simulink model "ControlsWithAutopilot"  (Simulink 8.5)
settings: Solver=ode45  StartTime=0.0  StopTime=10.0  RelTol=1e-3
undefined symbols (not defined in the file): ap, bias, sgn, sigbuilder_block
libraries: simulink x3
(part 1 of 2)
settings Model: Creator=mddavies  LastModifiedBy=teme
settings DataIOCC: SignalLoggingSaveFormat=Dataset
settings OptimizationCC: ExpressionDepthLimit=128
settings DebuggingCC: SolverPrmCheckMsg=warning  FcnCallInpInsideContextMsg=EnableAllAsError
settings GRTTargetCC: CombineOutputUpdateFcns=on  GRTInterface=off

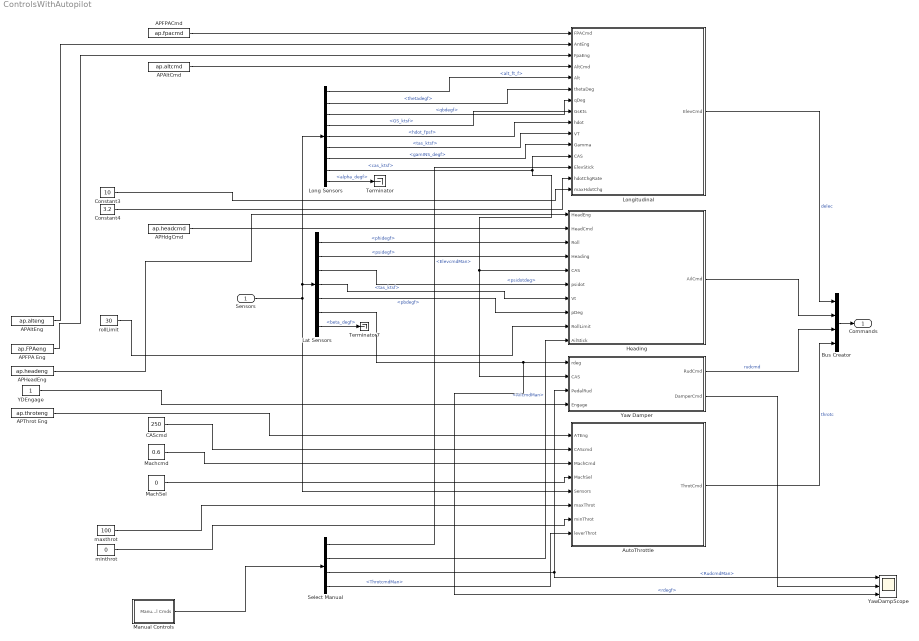
== system ControlsWithAutopilot ==
  Sensors : Inport  RequirementInfo={} %GIDa_0ce9b168_5661_42b0_b4cb_7d3faaf2df72
  APAltCmd : Constant  RequirementInfo={} %GIDa_8396ea73_c2c1_410d_8e72_0a2c2e115229  Value=ap.altcmd
  APAltEng : Constant  RequirementInfo={} %GIDa_7acdc276_5904_4f5d_a4d8_b7eafc22dcba  Value=ap.alteng  OutDataTypeStr=boolean
  APFPA Eng : Constant  RequirementInfo={} %GIDa_b6347d6f_b14e_46b8_b79f_c4482e372009  Value=ap.FPAeng  OutDataTypeStr=boolean
  "APFPACmd " : Constant  RequirementInfo={} %GIDa_f2a9802e_c9ff_44b4_9c39_101c70e3085f  Value=ap.fpacmd
  APHdgCmd : Constant  RequirementInfo={} %GIDa_ca348917_806b_4c73_b099_958ce531bbd5  Value=ap.headcmd
  APHeadEng : Constant  RequirementInfo={} %GIDa_019c8883_de5f_448b_a478_e0a40c975d97  Value=ap.headeng  OutDataTypeStr=boolean
  APThrot Eng : Constant  RequirementInfo={} %GIDa_c34ca1b2_b760_48cb_8815_eaf096d766de  Value=ap.throteng  OutDataTypeStr=boolean
  AutoThrottle : Subsystem  RequirementInfo={'other' '..\..\tcm_requirements.docx' '@Simulink_requirement_item_20' 'true' 'Auto Throttle' '' } %GIDa_9e91f8aa_3697_4e86_a547_8b20eda6b794
  Bus Creator : BusCreator  RequirementInfo={} %GIDa_5779fa34_87f2_4a60_8a6f_c75523d39478
  CAScmd : Constant  RequirementInfo={} %GIDa_47d34f1f_8d24_42cb_857b_a6284aa9b10f  Value=250
  Constant3 : Constant  RequirementInfo={} %GIDa_6046f9e1_21da_4401_862c_288f604e8689  Value=10
  Constant4 : Constant  RequirementInfo={} %GIDa_dee93be0_a932_4ef0_a207_8f7329b01ca5  Value=3.2
  Heading : Subsystem
  Lat Sensors : BusSelector  RequirementInfo={} %GIDa_c91152ab_38e9_465d_8eae_17f025af2b05  OutputSignals=phidegf,psidegf,EulerRates.psidotdeg,tas_ktsf,pbdegf,rdegf,beta_degf
  Long Sensors : BusSelector  RequirementInfo={} %GIDa_ce929a80_b046_4828_a008_4896c3439942  OutputSignals=alt_ft_f,thetadegf,qbdegf,GS_ktsf,hdot_fpsf,tas_ktsf,gamINS_degf,cas_ktsf,alpha_degf
  Longitudinal : Subsystem
  MachSel : Constant  RequirementInfo={} %GIDa_703eecf9_8ffd_4677_9df1_b11ad3ff81be  Value=0
  Machcmd : Constant  RequirementInfo={} %GIDa_a015b01e_abfd_4965_a258_bc3318cb77ef  Value=0.6
  Manual Controls : Subsystem
  Select Manual : BusSelector  RequirementInfo={} %GIDa_c52611af_90d4_4176_9d9c_eafcdc879716  OutputSignals=ElevcmdMan,AilcmdMan,RudcmdMan,ThrotcmdMan
  Terminator : Terminator
  Terminator7 : Terminator
      settings: RequirementInfo={} %GIDa_ea750fcf_3a35_4ca3_ba61_16c7ba83d83d
  YDEngage : Constant  RequirementInfo={} %GIDa_1b340559_9c71_403c_9901_bf0a93e2b9fd  SampleTime=-1
  Yaw Damper : Subsystem  RequirementInfo={'other' '..\..\tcm_requirements.docx' '@Simulink_requirement_item_19' 'true' 'Yaw Damper' '' } %GIDa_4d9fd165_a151_41ab_8542_450c342372eb
  YawDampScope : Scope  NumInputPorts=3
      settings: RequirementInfo={} %GIDa_7592f6f2_c7e8_4acc_8768_b20cb3da46c8  YMin=-5~-5~-5  YMax=5~5~5
  maxthrot : Constant  RequirementInfo={} %GIDa_230ab06c_3fb9_421e_bdda_8f032886ed67  Value=100  SampleTime=-1
  minthrot : Constant  RequirementInfo={} %GIDa_e24cf5cf_680d_403e_8bf4_a3705f2cf8ca  Value=0  SampleTime=-1
  rollLimit : Constant  RequirementInfo={} %GIDa_80188ac9_3eb7_4583_8db0_ebf7b7448de5  Value=30  SampleTime=-1
  Commands : Outport  RequirementInfo={} %GIDa_ba9bc9f0_2997_4cec_8a5a_2cb65716cddf
  wires:
  Lat Sensors/6 -> YawDampScope/3, Yaw Damper/1(rdeg)  "<rdegf>"
  AutoThrottle/1(ThrotCmd) -> Bus Creator/4  "throtc"
  Longitudinal/1(ElevCmd) -> Bus Creator/1  "delec"
  Bus Creator/1 -> Commands/1
  Heading/1(AilCmd) -> Bus Creator/2
  Sensors/1 -> Lat Sensors/1, Long Sensors/1, AutoThrottle/5(Sensors)
  Long Sensors/8 -> Yaw Damper/2(CAS), Heading/5(CAS), Longitudinal/12(CAS)  "<cas_ktsf>"
  Lat Sensors/7 -> Terminator7/1  "<beta_degf>"
  Select Manual/2 -> Heading/10(AilStick)  "<AilcmdMan>"
  Select Manual/3 -> YawDampScope/1, Yaw Damper/3(PedalRud)  "<RudcmdMan>"
  CAScmd/1 -> AutoThrottle/2(CAScmd)
  Select Manual/4 -> AutoThrottle/8(leverThrot)  "<ThrotcmdMan>"
  APAltEng/1 -> Longitudinal/2(AntEng)
  Machcmd/1 -> AutoThrottle/3(MachCmd)
  MachSel/1 -> AutoThrottle/4(MachSel)
  APHeadEng/1 -> Heading/1(HeadEng)
  APFPA Eng/1 -> Longitudinal/3(FpaEng)
  APThrot Eng/1 -> AutoThrottle/1(ATEng)
  APHdgCmd/1 -> Heading/2(HeadCmd)
  Long Sensors/9 -> Terminator/1  "<alpha_degf>"
  "APFPACmd "/1 -> Longitudinal/1(FPACmd)
  APAltCmd/1 -> Longitudinal/4(AltCmd)
  Long Sensors/1 -> Longitudinal/5(Alt)  "<alt_ft_f>"
  Long Sensors/2 -> Longitudinal/6(thetaDeg)  "<thetadegf>"
  Long Sensors/3 -> Longitudinal/7(qDeg)  "<qbdegf>"
  Long Sensors/4 -> Longitudinal/8(GsKts)  "<GS_ktsf>"
  Long Sensors/5 -> Longitudinal/9(hdot)  "<hdot_fpsf>"
  Long Sensors/6 -> Longitudinal/10(VT)  "<tas_ktsf>"
  Long Sensors/7 -> Longitudinal/11(Gamma)  "<gamINS_degf>"
  Lat Sensors/1 -> Heading/3(Roll)  "<phidegf>"
  Lat Sensors/2 -> Heading/4(Heading)  "<psidegf>"
  Lat Sensors/3 -> Heading/6(psidot)  "<psidotdeg>"
  Lat Sensors/4 -> Heading/7(Vt)  "<tas_ktsf>"
  Lat Sensors/5 -> Heading/8(pDeg)  "<pbdegf>"
  maxthrot/1 -> AutoThrottle/6(maxThrot)
  minthrot/1 -> AutoThrottle/7(minThrot)
  Select Manual/1 -> Longitudinal/13(ElevStick)  "<ElevcmdMan>"
  Yaw Damper/2(DamperCmd) -> YawDampScope/2
  Yaw Damper/1(RudCmd) -> Bus Creator/3  "rudcmd"
  Constant3/1 -> Longitudinal/15(maxHdotChg)
  Constant4/1 -> Longitudinal/14(hdotChgRate)
  YDEngage/1 -> Yaw Damper/4(Engage)
  rollLimit/1 -> Heading/9(RollLimit)
  Manual Controls/1(Manual Cmds) -> Select Manual/1

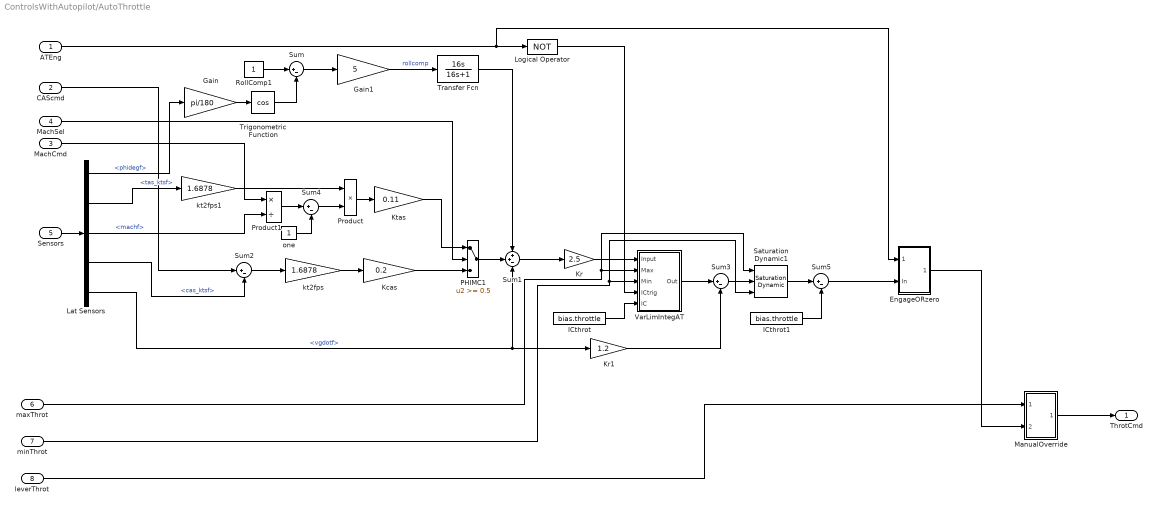
== system ControlsWithAutopilot/AutoThrottle ==
  ATEng : Inport  RequirementInfo={} %GIDa_2f45927d_6c28_4361_8173_5669474b9abd
  CAScmd : Inport  RequirementInfo={} %GIDa_92b5701d_5ed6_438c_8e94_843ad865eadf  Port=2
  MachCmd : Inport  RequirementInfo={} %GIDa_c26053c2_6b7f_4bf5_8f7d_768d0d646830  Port=3
  MachSel : Inport  RequirementInfo={} %GIDa_598b16f9_0dbe_4c96_859f_7e96536c1fb2  Port=4
  Sensors : Inport  RequirementInfo={} %GIDa_a55eff7f_fb2b_4f7a_a83b_479b402cff39  Port=5
  maxThrot : Inport  Port=6
  minThrot : Inport  Port=7
  leverThrot : Inport  Port=8
  EngageORzero : Subsystem
  Gain : Gain  RequirementInfo={} %GIDa_44ece66a_e9b1_47ae_9399_459633f82831  Gain=pi/180
  Gain1 : Gain  RequirementInfo={} %GIDa_5f70482a_3c80_415d_8392_528447a4813a  Gain=5
  ICthrot : Constant  RequirementInfo={} %GIDa_a96462ac_b28c_4fce_82e8_5e3952049bfb  Value=bias.throttle  SampleTime=-1
  ICthrot1 : Constant  RequirementInfo={} %GIDa_23dd534b_a590_436c_b15f_58e24838e8f2  Value=bias.throttle  SampleTime=-1
  Kcas : Gain  RequirementInfo={} %GIDa_1e6984b9_9479_49b0_970a_973f7c32edb7  Gain=0.2
  Kr : Gain  RequirementInfo={} %GIDa_18afb4c5_511e_47fb_85e5_bdfbcffb89de  Gain=2.5
  Kr1 : Gain  RequirementInfo={} %GIDa_9e9297b4_8c75_4533_a8dd_3891075538e5  Gain=1.2
  Ktas : Gain  RequirementInfo={} %GIDa_43c0fedf_b3e4_4e0f_a6fc_568c741b4ee2  Gain=0.11
  Lat Sensors : BusSelector  RequirementInfo={} %GIDa_4c677db3_3283_4698_82a6_69967aa56341  OutputSignals=phidegf,tas_ktsf,machf,cas_ktsf,vgdotf
  Logical Operator : Logic  RequirementInfo={} %GIDa_18e0a705_4fb5_4f14_a12b_8f6e047bc903  Operator=NOT  AllPortsSameDT=off  OutDataTypeStr=boolean
  ManualOverride : Subsystem
  PHIMC1 : Switch  RequirementInfo={} %GIDa_e2112eb0_c2db_4683_9846_bc0eb97a67f4  Threshold=0.5  SampleTime=0.02  SaturateOnIntegerOverflow=on
  Product : Product  RequirementInfo={} %GIDa_f2e51a99_89d7_4199_acd2_75b4a5a762fd  RndMeth=Zero
  Product1 : Product  RequirementInfo={} %GIDa_5c94e278_e588_4429_922d_3903b6601868  Inputs=*/  RndMeth=Zero
  RollComp1 : Constant  RequirementInfo={} %GIDa_8f810878_51f3_4d16_a407_aaec8ff4cd8a  SampleTime=-1
  Saturation Dynamic1 : simulink/Discontinuities/Saturation Dynamic  OutMin=[]  OutMax=[]  OutDataTypeStr=Inherit: Same as second input  OutDataType=sfix(16)  OutScaling=2^-10  DoSatur=off
  Sum : Sum  RequirementInfo={} %GIDa_9c88a12f_8eea_40db_a15a_aac24376aa7e  Inputs=|+-
  Sum1 : Sum  RequirementInfo={} %GIDa_fc0b036c_eb6d_4b0a_a40d_b7183183f1bc  Inputs=++-
  Sum2 : Sum  RequirementInfo={} %GIDa_95fcf8e7_99a7_46b3_9e41_77bfb2af0e6e  Inputs=|+-
  Sum3 : Sum  RequirementInfo={} %GIDa_0620e5c6_0d29_4c42_bdd5_2c680788712f  Inputs=|+-
  Sum4 : Sum  RequirementInfo={} %GIDa_a4cfd5ae_8cc7_4a4b_9229_0e28a225e0c7  Inputs=|+-
  Sum5 : Sum  RequirementInfo={} %GIDa_9cd0e9e4_7a0b_4a48_8c2a_57da4ad43678  Inputs=|+-
  Transfer Fcn : TransferFcn  RequirementInfo={} %GIDa_76b9b3a6_995f_4f78_b7a2_a7361be06aec  Numerator=[16 0]  Denominator=[16 1]
  Trigonometric Function : Trigonometry  RequirementInfo={} %GIDa_82d3b8e2_fba4_4fde_a324_6f5a5fa38b0e  Operator=cos
  VarLimIntegAT : Subsystem  RequirementInfo={} %GIDa_946bbead_442f_495f_943e_e8a8eb5a05a2
  kt2fps : Gain  RequirementInfo={} %GIDa_719dda5c_99e9_4155_8171_b1c9b5878f3a  Gain=1.6878
  kt2fps1 : Gain  RequirementInfo={} %GIDa_b06df2d8_ff63_4d20_83d9_1b3d18a391c7  Gain=1.6878
  one : Constant  RequirementInfo={} %GIDa_79530773_343c_40ed_88d6_a702a3c8b7d7  SampleTime=-1
  ThrotCmd : Outport  RequirementInfo={} %GIDa_10832092_f513_4063_bf4d_710db5c9192f
  wires:
  CAScmd/1 -> Sum2/1
  Sum2/1 -> kt2fps/1
  Sum1/1 -> Kr/1
  kt2fps/1 -> Kcas/1
  Kr/1 -> VarLimIntegAT/1(Input)
  Lat Sensors/5 -> Sum1/3, Kr1/1  "<vgdotf>"
  Kr1/1 -> Sum3/2
  Gain1/1 -> Transfer Fcn/1  "rollcomp"
  Sum/1 -> Gain1/1
  Trigonometric Function/1 -> Sum/2
  RollComp1/1 -> Sum/1
  Gain/1 -> Trigonometric Function/1
  Product1/1 -> Sum4/1
  one/1 -> Sum4/2
  Sum4/1 -> Product/2
  kt2fps1/1 -> Product/1
  Product/1 -> Ktas/1
  ICthrot/1 -> VarLimIntegAT/5(IC)
  Sum5/1 -> EngageORzero/2(In)
  ICthrot1/1 -> Sum5/2
  maxThrot/1 -> VarLimIntegAT/2(Max), Saturation Dynamic1/1
  minThrot/1 -> VarLimIntegAT/3(Min), Saturation Dynamic1/3
  VarLimIntegAT/1(Out) -> Sum3/1
  Sum3/1 -> Saturation Dynamic1/2
  Saturation Dynamic1/1 -> Sum5/1
  PHIMC1/1 -> Sum1/2
  Kcas/1 -> PHIMC1/3
  Ktas/1 -> PHIMC1/1
  Transfer Fcn/1 -> Sum1/1
  Sensors/1 -> Lat Sensors/1
  Lat Sensors/1 -> Gain/1  "<phidegf>"
  Lat Sensors/2 -> kt2fps1/1  "<tas_ktsf>"
  Lat Sensors/4 -> Sum2/2  "<cas_ktsf>"
  Logical Operator/1 -> VarLimIntegAT/4(ICtrig)
  ATEng/1 -> EngageORzero/1(Engage), Logical Operator/1
  MachSel/1 -> PHIMC1/2
  MachCmd/1 -> Product1/1
  Lat Sensors/3 -> Product1/2  "<machf>"
  leverThrot/1 -> ManualOverride/1(Man)
  ManualOverride/1(Out) -> ThrotCmd/1
  EngageORzero/1(Out) -> ManualOverride/2(Auto)

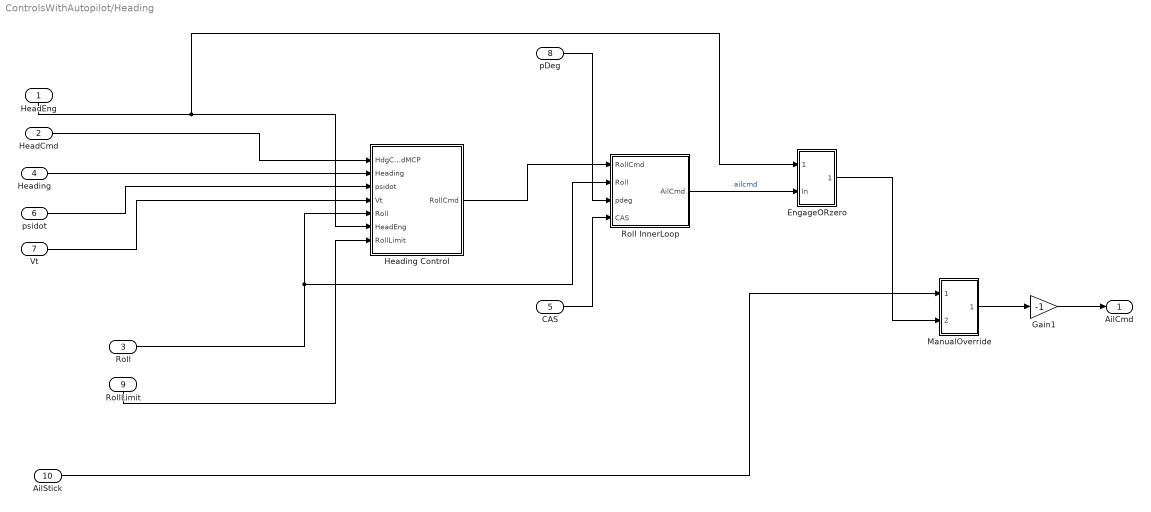
== system ControlsWithAutopilot/Heading ==
  HeadEng : Inport
  HeadCmd : Inport  Port=2
  Roll : Inport  Port=3
  Heading : Inport  Port=4
  CAS : Inport  Port=5
  psidot : Inport  Port=6
  Vt : Inport  Port=7
  pDeg : Inport  Port=8
  RollLimit : Inport  Port=9
  AilStick : Inport  Port=10
  EngageORzero : Subsystem
  Gain1 : Gain  RequirementInfo={} %GIDa_2f421c02_996e_46c9_ac2a_3c25b016b229  Gain=-1  SaturateOnIntegerOverflow=on  OutDataTypeStr=Inherit: Same as input  ParamDataTypeStr=Inherit: Same as input
  Heading Control : Subsystem  RequirementInfo={'other' '..\..\tcm_requirements.docx' '@Simulink_requirement_item_16' 'true' 'Heading Control' '' } %GIDa_911b8f78_7600_4481_9e93_a11b2a64dbe5
  ManualOverride : Subsystem
  Roll InnerLoop : Subsystem  RequirementInfo={'other' '..\..\tcm_requirements.docx' '@Simulink_requirement_item_18' 'true' 'Roll InnerLoop' '' } %GIDa_311280c1_10c2_4ab3_a776_5e785b9037f8
  AilCmd : Outport
  wires:
  pDeg/1 -> Roll InnerLoop/3(pdeg)
  Vt/1 -> Heading Control/4(Vt)
  psidot/1 -> Heading Control/3(psidot)
  Heading/1 -> Heading Control/2(Heading)
  Roll/1 -> Heading Control/5(Roll), Roll InnerLoop/2(Roll)
  Heading Control/1(RollCmd) -> Roll InnerLoop/1(RollCmd)
  Roll InnerLoop/1(AilCmd) -> EngageORzero/2(In)  "ailcmd"
  HeadCmd/1 -> Heading Control/1(HdgCmdMCP)
  HeadEng/1 -> EngageORzero/1(Engage), Heading Control/6(HeadEng)
  CAS/1 -> Roll InnerLoop/4(CAS)
  RollLimit/1 -> Heading Control/7(RollLimit)
  ManualOverride/1(Out) -> Gain1/1
  AilStick/1 -> ManualOverride/1(Man)
  Gain1/1 -> AilCmd/1
  EngageORzero/1(Out) -> ManualOverride/2(Auto)

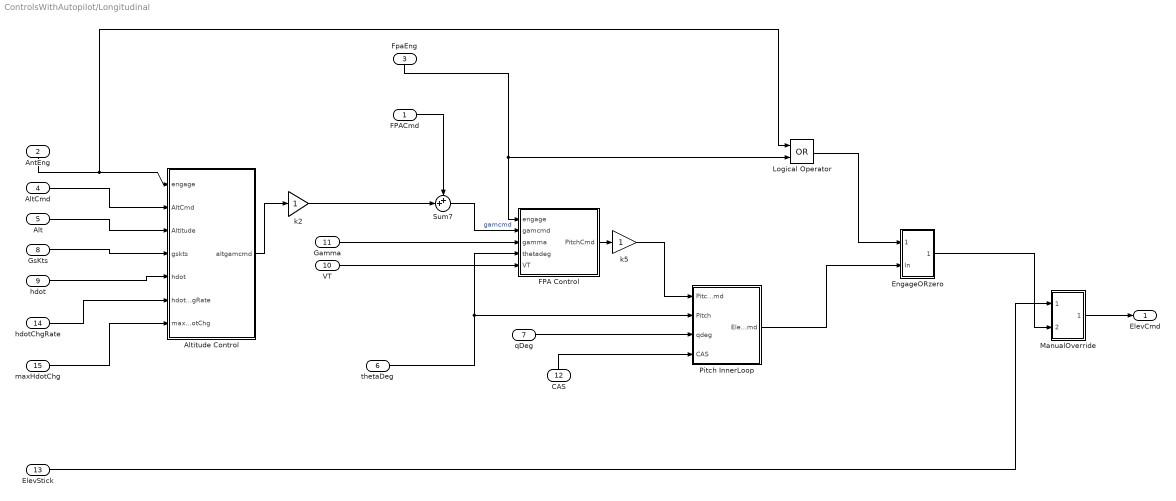
== system ControlsWithAutopilot/Longitudinal ==
  FPACmd : Inport
  AntEng : Inport  Port=2
  FpaEng : Inport  Port=3
  AltCmd : Inport  Port=4
  Alt : Inport  Port=5
  thetaDeg : Inport  Port=6
  qDeg : Inport  Port=7
  GsKts : Inport  Port=8
  hdot : Inport  Port=9
  VT : Inport  Port=10
  Gamma : Inport  Port=11
  CAS : Inport  Port=12
  ElevStick : Inport  Port=13
  hdotChgRate : Inport  Port=14
  maxHdotChg : Inport  Port=15
  Altitude Control : Subsystem  RequirementInfo={'other' '..\..\tcm_requirements.docx' '@Simulink_requirement_item_14' 'true' 'Altitude Control' '' } %GIDa_440f81f7_8b55_4c78_bea7_52c909831264
  EngageORzero : Subsystem
  FPA Control : Subsystem  RequirementInfo={'other' '..\..\tcm_requirements.docx' '@Simulink_requirement_item_15' 'true' 'FPA Control' '' } %GIDa_71e3e321_cc66_4d8a_a4f3_fd2e7f1fbaff
  Logical Operator : Logic  Operator=OR  AllPortsSameDT=off  OutDataTypeStr=boolean
  ManualOverride : Subsystem
  Pitch InnerLoop : Subsystem  RequirementInfo={'other' '..\..\tcm_requirements.docx' '@Simulink_requirement_item_17' 'true' 'Pitch InnerLoop' '' } %GIDa_fc56dd5e_d6cd_42fe_934f_e4aed2c76eb1
  Sum7 : Sum  RequirementInfo={} %GIDa_92495686_3877_4412_b19f_22e099e095ee  Inputs=++|
  k2 : Gain  RequirementInfo={} %GIDa_7e514706_5da4_4f1f_bf6c_0050dd9ce76d
  k5 : Gain  RequirementInfo={} %GIDa_b8b0ba7d_7fd3_4b03_b740_56530c3187c8
  ElevCmd : Outport
  wires:
  k2/1 -> Sum7/2
  Alt/1 -> Altitude Control/3(Altitude)
  thetaDeg/1 -> FPA Control/4(thetadeg), Pitch InnerLoop/2(Pitch)
  Gamma/1 -> FPA Control/3(gamma)
  AltCmd/1 -> Altitude Control/2(AltCmd)
  ManualOverride/1(Out) -> ElevCmd/1
  Altitude Control/1(altgamcmd) -> k2/1
  FPA Control/1(PitchCmd) -> k5/1
  hdot/1 -> Altitude Control/5(hdot)
  Sum7/1 -> FPA Control/2(gamcmd)  "gamcmd"
  qDeg/1 -> Pitch InnerLoop/3(qdeg)
  GsKts/1 -> Altitude Control/4(gskts)
  VT/1 -> FPA Control/5(VT)
  FPACmd/1 -> Sum7/1
  k5/1 -> Pitch InnerLoop/1(PitchCmd)
  FpaEng/1 -> Logical Operator/2, FPA Control/1(engage)
  CAS/1 -> Pitch InnerLoop/4(CAS)
  AntEng/1 -> Logical Operator/1, Altitude Control/1(engage)
  ElevStick/1 -> ManualOverride/1(Man)
  Pitch InnerLoop/1(ElevCmd) -> EngageORzero/2(In)
  EngageORzero/1(Out) -> ManualOverride/2(Auto)
  Logical Operator/1 -> EngageORzero/1(Engage)
  maxHdotChg/1 -> Altitude Control/7(maxHdotChg)
  hdotChgRate/1 -> Altitude Control/6(hdotChgRate)

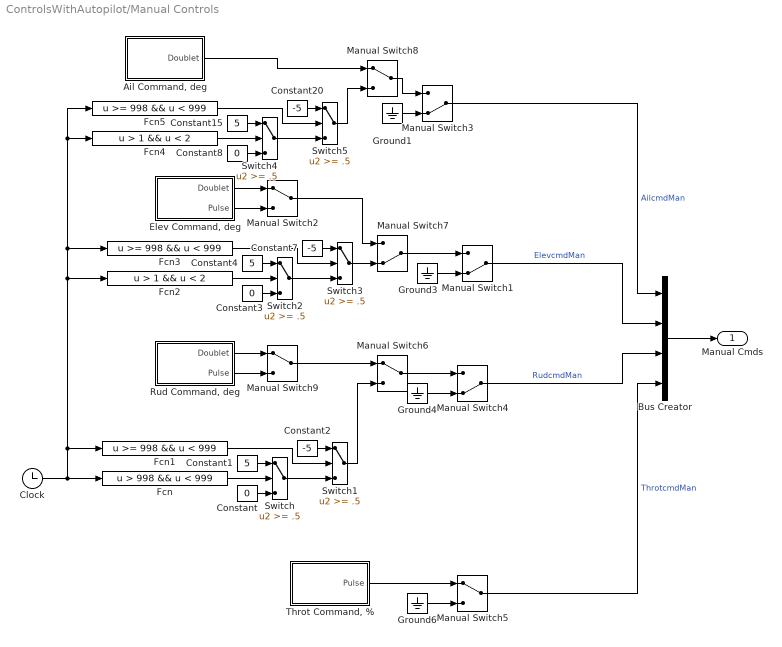
== system ControlsWithAutopilot/Manual Controls ==
  "Ail Command, deg" : Subsystem  Tag=STV Subsys  LoadFcn=sigbuilder_block('load');  StartFcn=sigbuilder_block('start');  StopFcn=sigbuilder_block('stop');  ClipboardFcn=sigbuilder_block('clipboard');  mask(Sigbuilder block){}
      mask help: Sigbuilder GUI
      mask init:
      | if ~strcmp(get_param(bdroot(gcbh),'SimulationStatus'),'stopped') tuvar = sigbuilder_block('maskInit'); end
      settings: CopyFcn=sigbuilder_block('copy');  DeleteFcn=sigbuilder_block('delete');  ModelCloseFcn=sigbuilder_block('modelClose');  PreSaveFcn=sigbuilder_block('preSave');  PauseFcn=sigbuilder_block('pause')  ContinueFcn=sigbuilder_block('continue')  NameChangeFcn=sigbuilder_block('namechange');  OpenFcn=sigbuilder_block('open',[20.16 261.12 550.08 400.32 ]);  CloseFcn=sigbuilder_block('close');
      mask Display: plot(0,0,100,100,[10,10,40,40,10],[80,20,20,80,80],[40,10],[50,50], [40,27,10],[65,72,56],[40,25,25,10],[28,28,43,43]);
  Bus Creator : BusCreator
  Clock : Clock
  Constant : Constant  Value=0
  Constant1 : Constant  Value=5
  Constant15 : Constant  Value=5
  Constant2 : Constant  Value=-5
  Constant20 : Constant  Value=-5
  Constant3 : Constant  Value=0
  Constant4 : Constant  Value=5
  Constant7 : Constant  Value=-5
  Constant8 : Constant  Value=0
  "Elev Command, deg" : Subsystem  Tag=STV Subsys  LoadFcn=sigbuilder_block('load');  StartFcn=sigbuilder_block('start');  StopFcn=sigbuilder_block('stop');  ClipboardFcn=sigbuilder_block('clipboard');  mask(Sigbuilder block){}
      mask help: Sigbuilder GUI
      mask init:
      | if ~strcmp(get_param(bdroot(gcbh),'SimulationStatus'),'stopped') tuvar = sigbuilder_block('maskInit'); end
      settings: CopyFcn=sigbuilder_block('copy');  DeleteFcn=sigbuilder_block('delete');  ModelCloseFcn=sigbuilder_block('modelClose');  PreSaveFcn=sigbuilder_block('preSave');  PauseFcn=sigbuilder_block('pause')  ContinueFcn=sigbuilder_block('continue')  NameChangeFcn=sigbuilder_block('namechange');  OpenFcn=sigbuilder_block('open',[550.08 198.72 550.08 400.32 ]);  CloseFcn=sigbuilder_block('close');
      mask Display: plot(0,0,100,100,[10,10,40,40,10],[80,20,20,80,80],[40,10],[50,50], [40,27,10],[65,72,56],[40,25,25,10],[28,28,43,43]);
  Fcn : Fcn  Expr=u > 998 && u < 999
  Fcn1 : Fcn  Expr=u >= 998 && u < 999
  Fcn2 : Fcn  Expr=u > 1 && u < 2
  Fcn3 : Fcn  Expr=u >= 998 && u < 999
  Fcn4 : Fcn  Expr=u > 1 && u < 2
  Fcn5 : Fcn  Expr=u >= 998 && u < 999
  Ground{1,3..4,6} (4 alike) : Ground
  Manual Switch{1,3..4,7} (4 alike) : ManualSwitch  CurrentSetting=0
  Manual Switch{2,5..6,8..9} (5 alike) : ManualSwitch
  "Rud Command, deg" : Subsystem  Tag=STV Subsys  LoadFcn=sigbuilder_block('load');  StartFcn=sigbuilder_block('start');  StopFcn=sigbuilder_block('stop');  ClipboardFcn=sigbuilder_block('clipboard');  mask(Sigbuilder block){}
      mask help: Sigbuilder GUI
      mask init:
      | if ~strcmp(get_param(bdroot(gcbh),'SimulationStatus'),'stopped') tuvar = sigbuilder_block('maskInit'); end
      settings: CopyFcn=sigbuilder_block('copy');  DeleteFcn=sigbuilder_block('delete');  ModelCloseFcn=sigbuilder_block('modelClose');  PreSaveFcn=sigbuilder_block('preSave');  PauseFcn=sigbuilder_block('pause')  ContinueFcn=sigbuilder_block('continue')  NameChangeFcn=sigbuilder_block('namechange');  OpenFcn=sigbuilder_block('open',[437.6 199.2 550.4 400 ]);  CloseFcn=sigbuilder_block('close');
      mask Display: plot(0,0,100,100,[10,10,40,40,10],[80,20,20,80,80],[40,10],[50,50], [40,27,10],[65,72,56],[40,25,25,10],[28,28,43,43]);
  Switch{,1..5} (6 alike) : Switch  Threshold=.5
  "Throt Command, %" : Subsystem  Tag=STV Subsys  LoadFcn=sigbuilder_block('load');  StartFcn=sigbuilder_block('start');  StopFcn=sigbuilder_block('stop');  ClipboardFcn=sigbuilder_block('clipboard');  mask(Sigbuilder block){}
      mask help: Sigbuilder GUI
      mask init:
      | if ~strcmp(get_param(bdroot(gcbh),'SimulationStatus'),'stopped') tuvar = sigbuilder_block('maskInit'); end
      settings: CopyFcn=sigbuilder_block('copy');  DeleteFcn=sigbuilder_block('delete');  ModelCloseFcn=sigbuilder_block('modelClose');  PreSaveFcn=sigbuilder_block('preSave');  PauseFcn=sigbuilder_block('pause')  ContinueFcn=sigbuilder_block('continue')  NameChangeFcn=sigbuilder_block('namechange');  OpenFcn=sigbuilder_block('open',[436.656 201.841 549.567 399.685 ]);  CloseFcn=sigbuilder_block('close');
      mask Display: plot(0,0,100,100,[10,10,40,40,10],[80,20,20,80,80],[40,10],[50,50], [40,27,10],[65,72,56],[40,25,25,10],[28,28,43,43]);
  Manual Cmds : Outport
  wires:
  Ground1/1 -> Manual Switch3/2
  Ground3/1 -> Manual Switch1/2
  "Elev Command, deg"/1(Doublet) -> Manual Switch2/1
  "Elev Command, deg"/2(Pulse) -> Manual Switch2/2
  Ground4/1 -> Manual Switch4/2
  Ground6/1 -> Manual Switch5/2
  "Throt Command, %"/1(Pulse) -> Manual Switch5/1
  Fcn/1 -> Switch/2
  Constant1/1 -> Switch/1
  Constant/1 -> Switch/3
  Switch/1 -> Switch1/3
  Constant2/1 -> Switch1/1
  Fcn1/1 -> Switch1/2
  Clock/1 -> Fcn/1, Fcn1/1, Fcn2/1, Fcn3/1, Fcn5/1, Fcn4/1
  Manual Switch6/1 -> Manual Switch4/1
  Switch1/1 -> Manual Switch6/2
  Fcn2/1 -> Switch2/2
  Constant4/1 -> Switch2/1
  Constant3/1 -> Switch2/3
  Switch2/1 -> Switch3/3
  Constant7/1 -> Switch3/1
  Fcn3/1 -> Switch3/2
  Manual Switch7/1 -> Manual Switch1/1
  Switch3/1 -> Manual Switch7/2
  Manual Switch2/1 -> Manual Switch7/1
  Fcn4/1 -> Switch4/2
  Constant15/1 -> Switch4/1
  Constant8/1 -> Switch4/3
  Switch4/1 -> Switch5/3
  Constant20/1 -> Switch5/1
  Fcn5/1 -> Switch5/2
  Manual Switch8/1 -> Manual Switch3/1
  Switch5/1 -> Manual Switch8/2
  "Ail Command, deg"/1(Doublet) -> Manual Switch8/1
  Manual Switch3/1 -> Bus Creator/1  "AilcmdMan"
  Manual Switch1/1 -> Bus Creator/2  "ElevcmdMan"
  Manual Switch4/1 -> Bus Creator/3  "RudcmdMan"
  Manual Switch5/1 -> Bus Creator/4  "ThrotcmdMan"
  Bus Creator/1 -> Manual Cmds/1
  "Rud Command, deg"/1(Doublet) -> Manual Switch9/1
  "Rud Command, deg"/2(Pulse) -> Manual Switch9/2
  Manual Switch9/1 -> Manual Switch6/1

== system ControlsWithAutopilot/Yaw Damper ==
  rdeg : Inport  RequirementInfo={} %GIDa_aab456ca_baa8_40be_af7c_3007e2406789
  CAS : Inport  RequirementInfo={} %GIDa_ffc3df4d_90ed_429c_9905_ba1d5e1c6104  Port=2
  PedalRud : Inport  Port=3
  Engage : Inport  Port=4
  EngageORzero : Subsystem
  Kcas : Lookup  RequirementInfo={} %GIDa_a54aaa82_92c8_4b54_937a_3aadc5cc777a  InputValues=[0 120 350 500]  Table=[1.0 1.0 0.3 0.3]
  Kr : Gain  RequirementInfo={} %GIDa_e1600aee_198d_416e_b040_c3f06ae50aaa  Gain=1.25
  ManualOverride : Subsystem
  Product : Product  RequirementInfo={} %GIDa_b93a6279_44c9_4030_b746_3332e584ca8b  RndMeth=Zero
  YD_wo : TransferFcn  RequirementInfo={} %GIDa_e4ecddaf_b3d8_4a89_aabe_57315209a16f  Numerator=[1 0]  Denominator=[1 10]
  RudCmd : Outport  RequirementInfo={} %GIDa_5d934514_ad75_43c8_8562_5e4d07d2a065
  DamperCmd : Outport  Port=2
  wires:
  rdeg/1 -> Kr/1
  CAS/1 -> Kcas/1
  Kcas/1 -> Product/2
  ManualOverride/1(Out) -> RudCmd/1
  Kr/1 -> YD_wo/1
  YD_wo/1 -> Product/1
  EngageORzero/1(Out) -> ManualOverride/2(Auto), DamperCmd/1
  PedalRud/1 -> ManualOverride/1(Man)
  Engage/1 -> EngageORzero/1(Engage)
  Product/1 -> EngageORzero/2(In)

== system ControlsWithAutopilot/AutoThrottle/EngageORzero ==
  Engage : Inport
  In : Inport  Port=2
  Logical Operator5 : Logic  RequirementInfo={} %GIDa_13e72d9c_1630_4494_8181_04ea596767a9  AllPortsSameDT=off  OutDataTypeStr=boolean
  Switch1 : Switch  RequirementInfo={} %GIDa_d89bdcfc_1e33_494f_b3fe_e13e317b4b5d  Threshold=0.5
  zero10 : Constant  RequirementInfo={} %GIDa_d1e784f7_2146_48f6_874a_0add9f175ac2
  zero9 : Constant  RequirementInfo={} %GIDa_df8b3a8b_00d1_4891_87af_e83379ed0682  Value=0
  Out : Outport
  wires:
  Engage/1 -> Logical Operator5/1
  zero10/1 -> Logical Operator5/2
  zero9/1 -> Switch1/3
  In/1 -> Switch1/1
  Logical Operator5/1 -> Switch1/2
  Switch1/1 -> Out/1

== system ControlsWithAutopilot/AutoThrottle/ManualOverride ==
  Man : Inport
  Auto : Inport  Port=2
  Switch1 : Switch  RequirementInfo={} %GIDa_99412258_89e8_4c84_a7a6_8adb3817b9de  Criteria=u2 ~= 0  Threshold=0.5
  Out : Outport
  wires:
  Man/1 -> Switch1/3, Switch1/2
  Auto/1 -> Switch1/1
  Switch1/1 -> Out/1

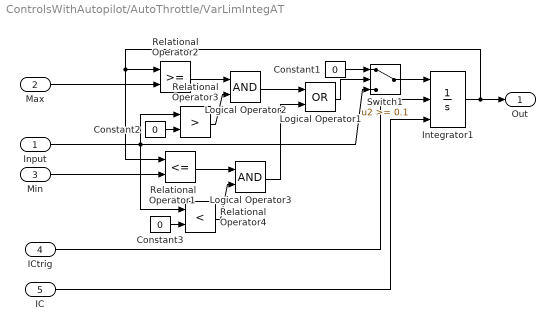
== system ControlsWithAutopilot/AutoThrottle/VarLimIntegAT ==
  Input : Inport  RequirementInfo={} %GIDa_91b38f96_ed38_45a6_8bb9_ff3fb81525df
  Max : Inport  RequirementInfo={} %GIDa_5200ce52_bb44_458c_9945_e382c2e773b4  Port=2
  Min : Inport  RequirementInfo={} %GIDa_600874e9_d5fd_4de5_b948_9284e9d56639  Port=3
  ICtrig : Inport  RequirementInfo={} %GIDa_af678c0a_424b_44b8_aa3a_3f303d846e8e  Port=4
  IC : Inport  RequirementInfo={} %GIDa_872b1a96_8436_4d34_8580_74ad3366301d  Port=5
  Constant1 : Constant  RequirementInfo={} %GIDa_bf704cc0_6bc9_4624_9fa4_e77befe43ee9  Value=0  SampleTime=-1
  Constant2 : Constant  RequirementInfo={} %GIDa_7032ed75_2ad3_41e5_9584_0891c369141c  Value=0  SampleTime=-1
  Constant3 : Constant  RequirementInfo={} %GIDa_f4367f96_4d82_41b7_8e43_0c6cec23a023  Value=0  SampleTime=-1
  Integrator1 : Integrator  RequirementInfo={} %GIDa_d4336f3d_c52f_4cf1_85ef_86b185e703b9  ExternalReset=level  InitialConditionSource=external
  Logical Operator1 : Logic  RequirementInfo={} %GIDa_53e2ecf2_1671_4b86_a4e6_7e9f03594f4a  Operator=OR
  Logical Operator2 : Logic  RequirementInfo={} %GIDa_f9639a17_73a7_4a19_b9c3_2b3e1bcf1152
  Logical Operator3 : Logic  RequirementInfo={} %GIDa_53705a9e_f0e6_4df8_b74a_51dda5b71ea0
  Relational Operator1 : RelationalOperator  RequirementInfo={} %GIDa_85cee0a0_d47b_41e2_b8dd_f48b296f5cf4  Operator=<=  InputSameDT=on
  Relational Operator2 : RelationalOperator  RequirementInfo={} %GIDa_74942223_cbc1_42b5_8e5e_e6b9112f9130  InputSameDT=on
  Relational Operator3 : RelationalOperator  RequirementInfo={} %GIDa_ea1202bb_7a42_4314_84fa_c36aa79c966a  Operator=>  InputSameDT=on
  Relational Operator4 : RelationalOperator  RequirementInfo={} %GIDa_c9e3adfb_bd3d_4cfe_9bd6_4a3fd1707fe2  Operator=<  InputSameDT=on
  Switch1 : Switch  RequirementInfo={} %GIDa_ed603307_5c4b_4569_8f05_95ce39b1df88  Threshold=0.1  SaturateOnIntegerOverflow=on  InputSameDT=on
  Out : Outport  RequirementInfo={} %GIDa_a7cb998d_eb28_45ce_8ac9_f1554f32fe4e
  wires:
  IC/1 -> Integrator1/3
  ICtrig/1 -> Integrator1/2
  Min/1 -> Relational Operator1/2
  Max/1 -> Relational Operator2/2
  Constant3/1 -> Relational Operator4/2
  Input/1 -> Switch1/3, Relational Operator3/1, Relational Operator4/1
  Logical Operator3/1 -> Logical Operator1/2
  Relational Operator4/1 -> Logical Operator3/2
  Relational Operator1/1 -> Logical Operator3/1
  Constant2/1 -> Relational Operator3/2
  Logical Operator2/1 -> Logical Operator1/1
  Relational Operator3/1 -> Logical Operator2/2
  Relational Operator2/1 -> Logical Operator2/1
  Logical Operator1/1 -> Switch1/2
  Integrator1/1 -> Relational Operator2/1, Relational Operator1/1, Out/1
  Switch1/1 -> Integrator1/1
  Constant1/1 -> Switch1/1

== system ControlsWithAutopilot/Heading/EngageORzero ==
  Engage : Inport
  In : Inport  Port=2
  Logical Operator5 : Logic  RequirementInfo={} %GIDa_7add67f6_200e_4459_8afc_a50a3802c341  AllPortsSameDT=off  OutDataTypeStr=boolean
  Switch1 : Switch  RequirementInfo={} %GIDa_a1777089_6daf_41d2_9e69_9356c4782e25  Threshold=0.5
  zero10 : Constant  RequirementInfo={} %GIDa_d889400f_b153_4cfc_a180_15b84145f1e0
  zero9 : Constant  RequirementInfo={} %GIDa_9027fd24_3b48_4acd_a774_517fb1aa3516  Value=0
  Out : Outport
  wires:
  Engage/1 -> Logical Operator5/1
  zero10/1 -> Logical Operator5/2
  zero9/1 -> Switch1/3
  In/1 -> Switch1/1
  Logical Operator5/1 -> Switch1/2
  Switch1/1 -> Out/1

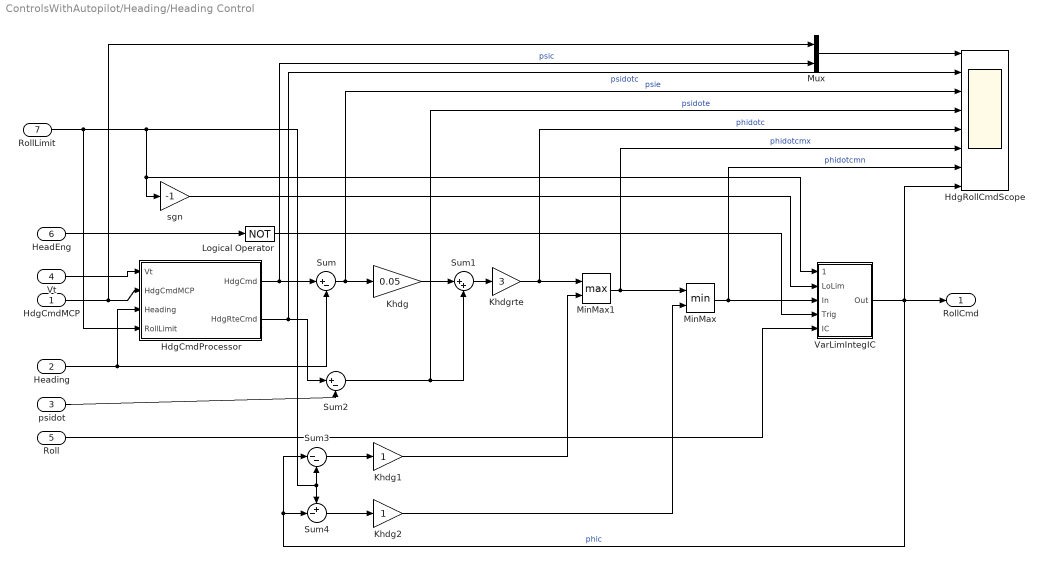
== system ControlsWithAutopilot/Heading/Heading Control ==
  HdgCmdMCP : Inport  RequirementInfo={} %GIDa_afcd05d1_a9dc_45a7_a8f8_7136ccc61726
  Heading : Inport  RequirementInfo={} %GIDa_19b80fe4_d265_482c_b709_18db80a7cdf3  Port=2
  psidot : Inport  RequirementInfo={} %GIDa_e421e82d_0cc7_4ad7_ac7a_9fb430d189d5  Port=3
  Vt : Inport  RequirementInfo={} %GIDa_9daf3e20_e00e_4f36_b534_d9747a241338  Port=4
  Roll : Inport  RequirementInfo={} %GIDa_8629ba77_a751_4097_af53_617eaa1017be  Port=5
  HeadEng : Inport  RequirementInfo={} %GIDa_dadb1310_2bf4_48cf_8970_85174d784ee3  Port=6
  RollLimit : Inport  Port=7
  HdgCmdProcessor : Subsystem  RequirementInfo={} %GIDa_3cb77e5f_f630_4f22_88a8_7528bfceb83f
  HdgRollCmdScope : Scope  NumInputPorts=8
      settings: RequirementInfo={} %GIDa_5fbe2135_fdf1_4f64_a179_faa1710ae21e  YMin=-30~-30~-10~-10~-4~-10~0~-5  YMax=30~30~10~10~4~10~1~5  SaveName=ScopeData7
  Khdg : Gain  RequirementInfo={} %GIDa_abf81b08_c210_4343_b4da_5a7e229caeb6  Gain=0.05
  Khdg1 : Gain  RequirementInfo={} %GIDa_7a7a35ca_24a5_4d20_bc30_55deea16462c
  Khdg2 : Gain  RequirementInfo={} %GIDa_57191899_7ee5_4454_897a_7009651ed5fb
  Khdgrte : Gain  RequirementInfo={} %GIDa_bcc6a420_18f3_43f0_aaa1_aaa1bbf90f64  Gain=3
  Logical Operator : Logic  RequirementInfo={} %GIDa_5ad405ac_0a88_4b96_aa0e_75483351ee25  Operator=NOT  AllPortsSameDT=off  OutDataTypeStr=boolean
  MinMax : MinMax  RequirementInfo={} %GIDa_4b9381d8_eb85_418b_a975_85846d5ca8c2  Inputs=2
  MinMax1 : MinMax  RequirementInfo={} %GIDa_b40e082d_0fb2_4088_baf4_e9a71be9bcc1  Function=max  Inputs=2
  Mux : Mux  RequirementInfo={} %GIDa_0e83f6c6_ae04_43dd_95fe_a79ec32b40e2  Inputs=2
  Sum : Sum  RequirementInfo={} %GIDa_b89885fc_f86c_4a50_8ce5_47d0488bdc1c  Inputs=|+-
  Sum1 : Sum  RequirementInfo={} %GIDa_40ec6862_b1f8_4f97_ae14_1eadabbceb30  Inputs=|++
  Sum2 : Sum  RequirementInfo={} %GIDa_307d6880_3ab8_4deb_90e0_d68f11d87c85  Inputs=|+-
  Sum3 : Sum  RequirementInfo={} %GIDa_ebb8b765_7f4a_435f_be61_680d3199141b  Inputs=|--
  Sum4 : Sum  RequirementInfo={} %GIDa_05638559_562a_476e_9e4c_91124434a43b  Inputs=+-|
  VarLimIntegIC : Subsystem  RequirementInfo={} %GIDa_7da7eaf5_9731_498e_9aad_b41279918004
  sgn : Gain  RequirementInfo={} %GIDa_84e2dc00_f2e5_41f4_89ce_c9fef234974f  Gain=-1
  RollCmd : Outport  RequirementInfo={} %GIDa_aa862f7f_5d4e_408f_b8c4_26b4ce96fbda
  wires:
  Heading/1 -> Sum/2, HdgCmdProcessor/3(Heading)
  HdgCmdProcessor/1(HdgCmd) -> Sum/1, Mux/2  "psic"
  Sum/1 -> Khdg/1, HdgRollCmdScope/3  "psie"
  Khdg/1 -> Sum1/1
  Sum2/1 -> Sum1/2, HdgRollCmdScope/4  "psidote"
  HdgCmdProcessor/2(HdgRteCmd) -> Sum2/1, HdgRollCmdScope/2  "psidotc"
  psidot/1 -> Sum2/2
  Vt/1 -> HdgCmdProcessor/1(Vt)
  HdgCmdMCP/1 -> HdgCmdProcessor/2(HdgCmdMCP), Mux/1
  VarLimIntegIC/1(Out) -> RollCmd/1, Sum3/1, Sum4/2, HdgRollCmdScope/8  "phic"
  RollLimit/1 -> HdgCmdProcessor/4(RollLimit), Sum4/1, Sum3/2, VarLimIntegIC/1(UpLim), sgn/1
  sgn/1 -> VarLimIntegIC/2(LoLim)
  Sum1/1 -> Khdgrte/1
  MinMax1/1 -> MinMax/1, HdgRollCmdScope/6  "phidotcmx"
  MinMax/1 -> VarLimIntegIC/3(In), HdgRollCmdScope/7  "phidotcmn"
  HeadEng/1 -> Logical Operator/1
  Sum3/1 -> Khdg1/1
  Sum4/1 -> Khdg2/1
  Khdg1/1 -> MinMax1/2
  Khdg2/1 -> MinMax/2
  Roll/1 -> VarLimIntegIC/5(IC)
  Khdgrte/1 -> MinMax1/1, HdgRollCmdScope/5  "phidotc"
  Logical Operator/1 -> VarLimIntegIC/4(Trig)
  Mux/1 -> HdgRollCmdScope/1

== system ControlsWithAutopilot/Heading/ManualOverride ==
  Man : Inport
  Auto : Inport  Port=2
  Switch1 : Switch  RequirementInfo={} %GIDa_5800ea93_45af_42da_974c_4cd975d0b8c8  Criteria=u2 ~= 0  Threshold=0.5
  Out : Outport
  wires:
  Man/1 -> Switch1/3, Switch1/2
  Auto/1 -> Switch1/1
  Switch1/1 -> Out/1

== system ControlsWithAutopilot/Heading/Roll InnerLoop ==
  note: orig =[0 60 140]
  note: orig = 0.25
  note: orig = 0.8
  RollCmd : Inport  RequirementInfo={} %GIDa_549f9d91_ca5c_4ec7_bf56_cf05f3793396
  Roll : Inport  RequirementInfo={} %GIDa_d885705c_af8c_4e18_b4d1_2f073687ea2c  Port=2
  pdeg : Inport  RequirementInfo={} %GIDa_ba7aa095_15b8_4f85_9051_8b947d28a24d  Port=3
  CAS : Inport  RequirementInfo={} %GIDa_defe4f55_1722_479a_b684_dc07a497c4ef  Port=4
  Kcas : Lookup  RequirementInfo={} %GIDa_a4bb01cf_3e83_4399_bf23_48aae96637bb  InputValues=[0 120 350 500]  Table=[1.0 1.0 0.3 0.3]
  Kphierr : Gain  RequirementInfo={} %GIDa_96c602a9_a07d_4519_9a2c_04c20a8c958d  Gain=0.5
  Product : Product  RequirementInfo={} %GIDa_6029a1e1_bbec_4e58_a2a6_3f9df62d6e90  RndMeth=Zero
  Roll_IL_scope : Scope  NumInputPorts=7
      settings: RequirementInfo={} %GIDa_ec5ee575_c049_4397_a5dd_5347629f97a6  YMin=-30~-30~-10~-10~-4~-10~0  YMax=30~30~10~10~4~10~1  SaveName=ScopeData5
  Sum : Sum  RequirementInfo={} %GIDa_6dd565f9_cc9c_463a_985b_c182e040d7fd  Inputs=|+-
  Sum1 : Sum  RequirementInfo={} %GIDa_02561aa6_0360_4e6c_b76e_5dde7f2ab3b1  Inputs=|+-
  rollrate_IL : ZeroPole  RequirementInfo={} %GIDa_636569be_bc7e_4244_84a4_4a62b7fc0808  Zeros=0  Poles=-0.5  Gain=0.00645
  AilCmd : Outport  RequirementInfo={} %GIDa_cd7ddcd8_c7c7_43e2_be4e_2c0bb3f4c702
  wires:
  Product/1 -> AilCmd/1, Roll_IL_scope/6  "ailcmd"
  Kcas/1 -> Product/2, Roll_IL_scope/7  "kcas"
  Sum1/1 -> Product/1
  CAS/1 -> Kcas/1
  rollrate_IL/1 -> Sum1/2, Roll_IL_scope/5  "pdegwo"
  pdeg/1 -> rollrate_IL/1, Roll_IL_scope/4  "pdeg"
  Kphierr/1 -> Sum1/1
  Roll/1 -> Sum/2, Roll_IL_scope/2  "roll"
  Sum/1 -> Kphierr/1, Roll_IL_scope/3  "rollerr"
  RollCmd/1 -> Sum/1, Roll_IL_scope/1  "rollcmd"

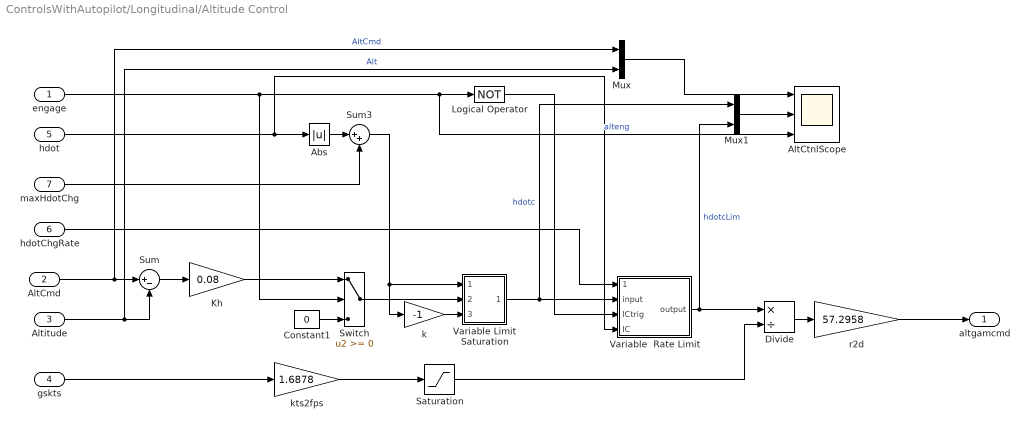
== system ControlsWithAutopilot/Longitudinal/Altitude Control ==
  engage : Inport  RequirementInfo={} %GIDa_92edc9e2_4cfd_4b16_8fee_8b94964575da
  AltCmd : Inport  RequirementInfo={} %GIDa_edbc7e5c_23e1_4d8f_98c5_e2d77895a510  Port=2
  Altitude : Inport  RequirementInfo={} %GIDa_01b40abf_ece8_4194_aeed_7639b2f9d320  Port=3
  gskts : Inport  RequirementInfo={} %GIDa_49aaf918_ec6b_4cc9_bdad_efb02f39ea3b  Port=4
  hdot : Inport  RequirementInfo={} %GIDa_f8353919_6ca2_40ed_9884_9c34b61b1365  Port=5
  hdotChgRate : Inport  Port=6
  maxHdotChg : Inport  Port=7
  Abs : Abs  RequirementInfo={} %GIDa_1391aa7c_5846_4be5_914e_111d8f2c4215  SaturateOnIntegerOverflow=on
  AltCtnlScope : Scope  NumInputPorts=3
      settings: RequirementInfo={} %GIDa_baad481c_a27b_41ac_bf32_d6e1a7f2cfe1  TimeRange=30  YMin=10000~-5~0  YMax=10200~15~1  SaveName=ScopeData3
  Constant1 : Constant  RequirementInfo={} %GIDa_566c4b52_316f_4d36_82bb_fb65e53f78d2  Value=0
  Divide : Product  RequirementInfo={} %GIDa_b9d1a3fe_7e00_46b2_9426_cf952dcaf391  Inputs=*/
  Kh : Gain  RequirementInfo={} %GIDa_de6b2d53_b3f4_42e2_83e9_439be9ccc299  Gain=0.08
  Logical Operator : Logic  RequirementInfo={} %GIDa_921e6188_0ac2_4a9c_befc_5c7a6835e9e6  Operator=NOT
  Mux : Mux  RequirementInfo={} %GIDa_68aa779e_2c07_4c3b_9ca1_0ecb3161e49a  Inputs=2
  Mux1 : Mux  RequirementInfo={} %GIDa_0a0909f8_d09a_4568_9828_3f29982a74b3  Inputs=2
  Saturation : Saturate  RequirementInfo={} %GIDa_77166b67_e163_40e1_b7e4_7e7410a56d29  UpperLimit=1000  LowerLimit=0.0001
  Sum : Sum  RequirementInfo={} %GIDa_d94a0856_9d8d_4fca_8b77_5f1cf21c0c3a  Inputs=|+-
  Sum3 : Sum  RequirementInfo={} %GIDa_3ee7802b_411f_4586_886f_8bdef6cfccb9  Inputs=|++  SaturateOnIntegerOverflow=on  InputSameDT=on  OutDataTypeStr=Inherit: Same as first input
  Switch : Switch  RequirementInfo={} %GIDa_64af29d5_be60_4de8_bcf5_833ab8e70f35
  Variable  Rate Limit : Subsystem  RequirementInfo={} %GIDa_7d0e1926_4469_4591_916e_2bb88ddee008
  Variable Limit Saturation : Subsystem  RequirementInfo={} %GIDa_0b931211_59c1_4508_94b8_12d4cca2cb6b
  k : Gain  RequirementInfo={} %GIDa_65a0c0b6_6e9b_4a97_b326_1d79079cc625  Gain=-1
  kts2fps : Gain  RequirementInfo={} %GIDa_a49848e7_9841_44de_8ec7_08f1ed28d1e0  Gain=1.6878
  r2d : Gain  RequirementInfo={} %GIDa_934ba914_aaac_471d_9b5e_a120031a3853  Gain=57.2958
  altgamcmd : Outport  RequirementInfo={} %GIDa_3c331913_004d_4e8f_a0a1_b052c80c7670
  wires:
  Sum/1 -> Kh/1
  AltCmd/1 -> Sum/1, Mux/1  "AltCmd"
  Altitude/1 -> Sum/2, Mux/2  "Alt"
  hdot/1 -> Abs/1, Variable  Rate Limit/4(IC)
  Abs/1 -> Sum3/1
  maxHdotChg/1 -> Sum3/2
  k/1 -> Variable Limit Saturation/3(Lo_lim)
  Sum3/1 -> k/1, Variable Limit Saturation/1(up_lim)
  engage/1 -> Switch/2, Logical Operator/1, AltCtnlScope/3  "alteng"
  gskts/1 -> kts2fps/1
  Divide/1 -> r2d/1
  r2d/1 -> altgamcmd/1
  Logical Operator/1 -> Variable  Rate Limit/3(ICtrig)
  Variable Limit Saturation/1(Out1) -> Variable  Rate Limit/2(input), Mux1/1  "hdotc"
  hdotChgRate/1 -> Variable  Rate Limit/1(ratelim)
  Variable  Rate Limit/1(output) -> Divide/1, Mux1/2  "hdotcLim"
  kts2fps/1 -> Saturation/1
  Saturation/1 -> Divide/2
  Switch/1 -> Variable Limit Saturation/2(SigIn)
  Kh/1 -> Switch/1
  Constant1/1 -> Switch/3
  Mux/1 -> AltCtnlScope/1
  Mux1/1 -> AltCtnlScope/2

== system ControlsWithAutopilot/Longitudinal/EngageORzero ==
  Engage : Inport
  In : Inport  Port=2
  Logical Operator5 : Logic  RequirementInfo={} %GIDa_2faaa958_fdd5_4161_8224_87bc655595ec  AllPortsSameDT=off  OutDataTypeStr=boolean
  Switch1 : Switch  RequirementInfo={} %GIDa_cd8505b1_f38c_41a3_a83c_5e083797b181  Threshold=0.5
  zero10 : Constant  RequirementInfo={} %GIDa_596a5899_ba53_4c37_8272_7211e27ddf24
  zero9 : Constant  RequirementInfo={} %GIDa_b5c8c028_3d9d_45c0_afd9_41cf87627ef7  Value=0
  Out : Outport
  wires:
  Engage/1 -> Logical Operator5/1
  zero10/1 -> Logical Operator5/2
  zero9/1 -> Switch1/3
  In/1 -> Switch1/1
  Logical Operator5/1 -> Switch1/2
  Switch1/1 -> Out/1

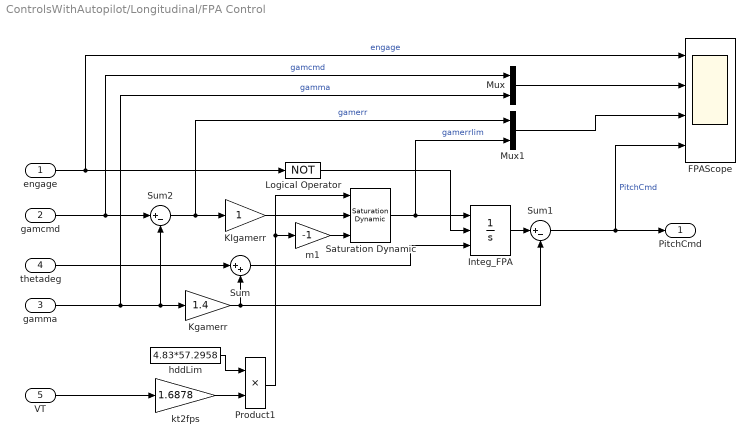
== system ControlsWithAutopilot/Longitudinal/FPA Control ==
  engage : Inport  RequirementInfo={} %GIDa_4330a6b4_8fd7_4be4_8132_0a5a51cb5321
  gamcmd : Inport  RequirementInfo={} %GIDa_72bd14a4_cf4e_4ddf_9979_bc189fd4e864  Port=2
  gamma : Inport  RequirementInfo={} %GIDa_07a290a4_e9be_4e9c_ae2b_d72f5ca4cb2b  Port=3
  thetadeg : Inport  RequirementInfo={} %GIDa_6ddd8d11_1197_4928_a2bc_231a82446ee7  Port=4
  VT : Inport  RequirementInfo={} %GIDa_a0a43ff9_fad6_4fc8_a8cd_c357b3dfb673  Port=5
  FPAScope : Scope  NumInputPorts=4
      settings: RequirementInfo={} %GIDa_08c55925_5efe_4d90_b09d_0072cafa98d7  YMin=-1~-5~-2~-5  YMax=2~5~2~10  SaveName=ScopeData12
  Integ_FPA : Integrator  RequirementInfo={} %GIDa_51acd94e_b58d_4d17_b07c_0b9ac17c0faa  ExternalReset=level  InitialConditionSource=external  IgnoreLimit=on
  KIgamerr : Gain  RequirementInfo={} %GIDa_08963e9e_c311_47c8_a63e_11cc7c9fb2d8
  Kgamerr : Gain  RequirementInfo={} %GIDa_3495b1a6_277d_4a6c_aa4f_649fc83b9092  Gain=1.4
  Logical Operator : Logic  RequirementInfo={} %GIDa_eba75fd0_479d_4894_b4e0_0ecea241815c  Operator=NOT  AllPortsSameDT=off  OutDataTypeStr=boolean
  Mux : Mux  RequirementInfo={} %GIDa_ae1e9d70_29ff_4004_97f5_396f2626ff0e  Inputs=2
  Mux1 : Mux  RequirementInfo={} %GIDa_b657458f_9c9c_48b1_af95_f550cfeae5f6  Inputs=2
  Product1 : Product  RequirementInfo={} %GIDa_bb863780_5e58_4e21_8791_e7a2c94dd786  RndMeth=Zero
  Saturation Dynamic : simulink/Discontinuities/Saturation Dynamic  OutMin=[]  OutMax=[]  OutDataTypeStr=Inherit: Same as second input  OutDataType=fixdt(1, 16)  OutScaling=2^-10  DoSatur=off
  Sum : Sum  RequirementInfo={} %GIDa_494c7255_4427_4dad_a3c1_4aee399936eb  Inputs=|++
  Sum1 : Sum  RequirementInfo={} %GIDa_93359946_60e9_438e_99e8_9beddee58b77  Inputs=|+-
  Sum2 : Sum  RequirementInfo={} %GIDa_c5e9feb7_f19d_4066_9b64_2fe045a465c2  Inputs=|+-
  hddLim : Constant  RequirementInfo={} %GIDa_1bf124ef_f3a0_4770_a704_52ef6436d4b5  Value=4.83*57.2958
  kt2fps : Gain  RequirementInfo={} %GIDa_c7ee5a6f_140d_48a3_b5c5_8ced7bef0603  Gain=1.6878
  m1 : Gain  RequirementInfo={} %GIDa_3e310fb8_58d1_4ad2_a1bc_b1914379a108  Gain=-1
  PitchCmd : Outport  RequirementInfo={} %GIDa_7e56bb7b_bd21_4466_8889_6a6d9858a2da
  wires:
  Sum1/1 -> PitchCmd/1, FPAScope/4  "PitchCmd"
  Kgamerr/1 -> Sum1/2, Sum/2
  Integ_FPA/1 -> Sum1/1
  gamma/1 -> Kgamerr/1, Sum2/2, Mux/2  "gamma"
  thetadeg/1 -> Sum/1
  Sum/1 -> Integ_FPA/3
  engage/1 -> Logical Operator/1, FPAScope/1  "engage"
  Logical Operator/1 -> Integ_FPA/2
  kt2fps/1 -> Product1/2
  hddLim/1 -> Product1/1
  Product1/1 -> Saturation Dynamic/1, m1/1
  VT/1 -> kt2fps/1
  Saturation Dynamic/1 -> Integ_FPA/1, Mux1/2  "gamerrlim"
  KIgamerr/1 -> Saturation Dynamic/2
  m1/1 -> Saturation Dynamic/3
  Sum2/1 -> KIgamerr/1, Mux1/1  "gamerr"
  gamcmd/1 -> Sum2/1, Mux/1  "gamcmd"
  Mux/1 -> FPAScope/2
  Mux1/1 -> FPAScope/3

== system ControlsWithAutopilot/Longitudinal/ManualOverride ==
  Man : Inport
  Auto : Inport  Port=2
  Switch1 : Switch  RequirementInfo={} %GIDa_891c72b6_c029_43c0_848a_219761f8f015  Criteria=u2 ~= 0  Threshold=0.5
  Out : Outport
  wires:
  Man/1 -> Switch1/3, Switch1/2
  Auto/1 -> Switch1/1
  Switch1/1 -> Out/1

== system ControlsWithAutopilot/Longitudinal/Pitch InnerLoop ==
  PitchCmd : Inport  RequirementInfo={} %GIDa_e681796d_a620_4c95_b4ed_ba3232dc70a2
  Pitch : Inport  RequirementInfo={} %GIDa_6f4baf24_a090_49e6_89b2_2ff3bd4fd377  Port=2
  qdeg : Inport  RequirementInfo={} %GIDa_13210493_e26c_4a14_89fc_8ad0299ca616  Port=3
  CAS : Inport  RequirementInfo={} %GIDa_e1a07f62_5dbf_46dc_bc2c_c2998ea01de8  Port=4
  Kcas : Lookup  RequirementInfo={} %GIDa_b4066843_ddd1_46cc_9bab_4de3e3ab273c  InputValues=[0 120 350 500]  Table=[1.0 1.0 0.3 0.3]
  Kpitch : Gain  RequirementInfo={} %GIDa_4a392bdb_3184_422c_b598_a156d3e8b02c  Gain=2
  Kwo : Gain  RequirementInfo={} %GIDa_6174b3c5_b132_42d6_a380_7a86f841c8e6  Gain=0.5
  Mux : Mux  RequirementInfo={} %GIDa_93279ee0_cc4a_4a25_b0b1_b731353743b0  Inputs=2
  PitchScope : Scope  NumInputPorts=6
      settings: RequirementInfo={} %GIDa_5646223d_16bd_44bf_9f51_c97977b5f9c0  YMin=-2~-2~-2~-20~-20~0  YMax=10~2~2~20~20~1.2  SaveName=ScopeData11
  Product : Product  RequirementInfo={} %GIDa_ee2099f1_df06_4fc6_bf9b_0b7652de3a20  RndMeth=Zero
  Sum : Sum  RequirementInfo={} %GIDa_6e966264_2a04_4ed3_91bc_90c4039fd9a0  Inputs=|+-
  Sum1 : Sum  RequirementInfo={} %GIDa_5254d09e_07d7_42ec_bb70_93117997e359  Inputs=|-+
  Transfer Fcn : TransferFcn  RequirementInfo={} %GIDa_3bfe3d6e_47ed_45cd_9b22_d5337598ae49  Numerator=[16 0]  Denominator=[16 1]
  ElevCmd : Outport  RequirementInfo={} %GIDa_133d9978_a863_4cc3_b149_7ebb5beb5068
  wires:
  Sum/1 -> Kpitch/1, PitchScope/2  "Pitcherror"
  Pitch/1 -> Sum/2, Mux/2
  Kpitch/1 -> Sum1/1
  qdeg/1 -> Transfer Fcn/1
  Transfer Fcn/1 -> Kwo/1
  CAS/1 -> Kcas/1
  Sum1/1 -> Product/1, PitchScope/4  "dec"
  Kcas/1 -> Product/2, PitchScope/6  "Kcas"
  Product/1 -> ElevCmd/1, PitchScope/5  "elevcmd"
  Kwo/1 -> Sum1/2, PitchScope/3  "qdegwo"
  PitchCmd/1 -> Sum/1, Mux/1  "Pitchcmd"
  Mux/1 -> PitchScope/1

== system ControlsWithAutopilot/Manual Controls/Ail Command, deg ==
  Demux : Demux  Tag=STV Demux  Outputs=1
  FromWs : FromWorkspace  Tag=STV FromWs  VariableName=tuvar  SampleTime=0  SigBuilderData=DataTag0  VnvData=DataTag1
      SigBuilderData=|
      | common.afterFinalStr = 'Extrapolate'
      | common.sampleTime = 0
      | dataSet.timeRange = [0 10]
      | dataSet.name = 'Group 1'
      | sbobj.Groups.Name = 'Group 1'
      | sbobj.Groups.Signals.Name = 'Doublet'
      | sbobj.Groups.Signals.XData = [0 1 1 2 2 2.98 2.98 10]
      | sbobj.Groups.Signals.YData = [0 0 5 5 -5 -5 0 0]
  Doublet : Outport  Tag=STV Outport
  wires:
  FromWs/1 -> Demux/1
  Demux/1 -> Doublet/1

== system ControlsWithAutopilot/Manual Controls/Elev Command, deg ==
  Demux : Demux  Tag=STV Demux  Outputs=2
  FromWs : FromWorkspace  Tag=STV FromWs  VariableName=tuvar  SampleTime=0  SigBuilderData=DataTag2  VnvData=DataTag3
      SigBuilderData=|
      | common.afterFinalStr = 'Extrapolate'
      | common.sampleTime = 0
      | dataSet.timeRange = [0 10]
      | dataSet.name = 'Group 1'
      | sbobj.Groups.Name = 'Group 1'
      | sbobj.Groups.Signals(1).Name = 'Doublet'
      | sbobj.Groups.Signals(1).XData = [0 1 1 2 2 3 3 10]
      | sbobj.Groups.Signals(1).YData = [0 0 5 5 -5 -5 0 0]
      | sbobj.Groups.Signals(2).Name = 'Pulse'
      | sbobj.Groups.Signals(2).XData = [0 1 1 2 2 10]
      | sbobj.Groups.Signals(2).YData = [0 0 1 1 0 0]
  Doublet : Outport  Tag=STV Outport
  Pulse : Outport  Tag=STV Outport  Port=2
  wires:
  Demux/1 -> Doublet/1
  FromWs/1 -> Demux/1
  Demux/2 -> Pulse/1

== system ControlsWithAutopilot/Manual Controls/Rud Command, deg ==
  Demux : Demux  Tag=STV Demux  Outputs=2
  FromWs : FromWorkspace  Tag=STV FromWs  VariableName=tuvar  SampleTime=0  SigBuilderData=DataTag4  VnvData=DataTag5
      SigBuilderData=|
      | common.afterFinalStr = 'Extrapolate'
      | common.sampleTime = 0
      | dataSet.timeRange = [0 10]
      | dataSet.name = 'Group 1'
      | sbobj.Groups.Name = 'Group 1'
      | sbobj.Groups.Signals(1).Name = 'Doublet'
      | sbobj.Groups.Signals(1).XData = [0 1 1 2 2 3 3 10]
      | sbobj.Groups.Signals(1).YData = [0 0 1 1 -1 -1 0 0]
      | sbobj.Groups.Signals(2).Name = 'Pulse'
      | sbobj.Groups.Signals(2).XData = [0 1 1 2 2 10]
      | sbobj.Groups.Signals(2).YData = [0 0 1 1 0 0]
  Doublet : Outport  Tag=STV Outport
  Pulse : Outport  Tag=STV Outport  Port=2
  wires:
  Demux/1 -> Doublet/1
  FromWs/1 -> Demux/1
  Demux/2 -> Pulse/1

== system ControlsWithAutopilot/Manual Controls/Throt Command, % ==
  Demux : Demux  Tag=STV Demux  Outputs=1
  FromWs : FromWorkspace  Tag=STV FromWs  VariableName=tuvar  SampleTime=0  SigBuilderData=DataTag6  VnvData=DataTag7
      SigBuilderData=|
      | common.afterFinalStr = 'Extrapolate'
      | common.sampleTime = 0
      | dataSet.timeRange = [0 100]
      | dataSet.name = 'Group 1'
      | sbobj.Groups.Name = 'Group 1'
      | sbobj.Groups.Signals.Name = 'Pulse'
      | sbobj.Groups.Signals.XData = [0 5 5 90.2 90.2 100]
      | sbobj.Groups.Signals.YData = [0 0 1 1 0 0]
      | sbobj.Groups.TimeRange = [0 100]
  Pulse : Outport  Tag=STV Outport
  wires:
  FromWs/1 -> Demux/1
  Demux/1 -> Pulse/1

== system ControlsWithAutopilot/Yaw Damper/EngageORzero ==
  Engage : Inport
  In : Inport  Port=2
  Logical Operator5 : Logic  RequirementInfo={} %GIDa_039f8944_4af0_4d9a_b296_dc63f4fb9b24  AllPortsSameDT=off  OutDataTypeStr=boolean
  Switch1 : Switch  RequirementInfo={} %GIDa_5a57b0db_bac7_4f14_9c86_f79c8d73773a  Threshold=0.5
  zero10 : Constant  RequirementInfo={} %GIDa_459066bd_0987_4218_99ad_2fd246291f08
  zero9 : Constant  RequirementInfo={} %GIDa_11be025e_2612_434d_af1e_162a733bf0cc  Value=0
  Out : Outport
  wires:
  Engage/1 -> Logical Operator5/1
  zero10/1 -> Logical Operator5/2
  zero9/1 -> Switch1/3
  In/1 -> Switch1/1
  Logical Operator5/1 -> Switch1/2
  Switch1/1 -> Out/1

== system ControlsWithAutopilot/Yaw Damper/ManualOverride ==
  Man : Inport
  Auto : Inport  Port=2
  Switch1 : Switch  RequirementInfo={} %GIDa_c20200e4_a463_47a4_8bca_86ae3712d2e3  Criteria=u2 ~= 0  Threshold=0.5
  Out : Outport
  wires:
  Man/1 -> Switch1/3, Switch1/2
  Auto/1 -> Switch1/1
  Switch1/1 -> Out/1

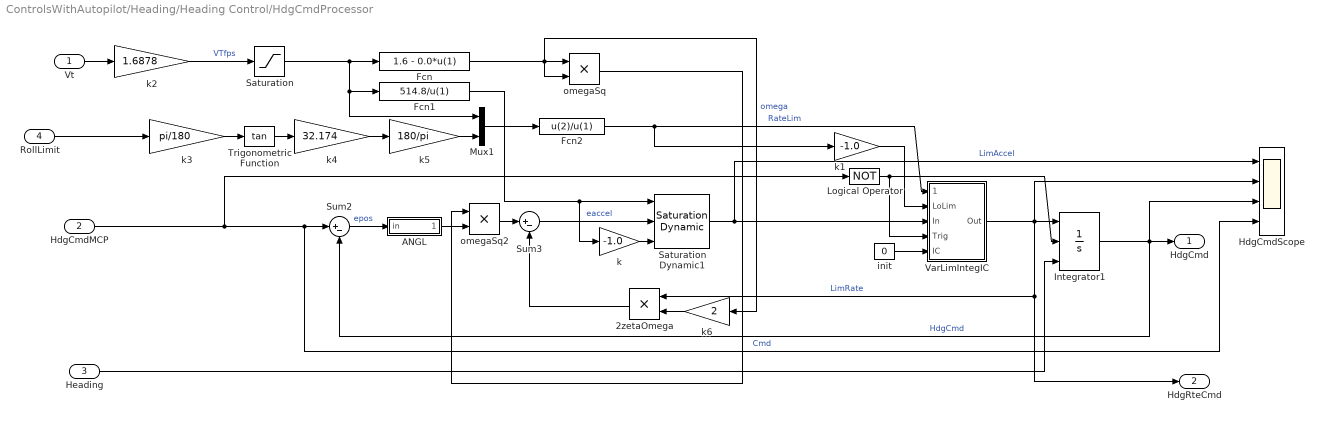
== system ControlsWithAutopilot/Heading/Heading Control/HdgCmdProcessor ==
  Vt : Inport  RequirementInfo={} %GIDa_aea371ad_7692_43c3_9333_237397a7088d
  HdgCmdMCP : Inport  RequirementInfo={} %GIDa_62146feb_aace_4fc2_8116_9e6cd7e3722f  Port=2
  Heading : Inport  RequirementInfo={} %GIDa_2367d888_2282_4a9b_9dc0_ce749bdb20fa  Port=3
  RollLimit : Inport  Port=4
  2zetaOmega : Product  RequirementInfo={} %GIDa_f321de1d_2313_4525_97dc_b8d5cf0673a7  RndMeth=Zero
  ANGL : Subsystem  RequirementInfo={} %GIDa_a65114d8_8cfa_43a6_b93e_efba84d5b466
  Fcn : Fcn  RequirementInfo={} %GIDa_4531d45e_6cbe_48a3_a177_15bd19e92740  Expr=1.6 - 0.0*u(1)
  Fcn1 : Fcn  RequirementInfo={} %GIDa_6e2df688_d84a_49b7_8178_2e4e2167c90a  Expr=514.8/u(1)
  Fcn2 : Fcn  RequirementInfo={} %GIDa_0806e265_28c4_47b9_a883_58ecb6812137  Expr=u(2)/u(1)
  HdgCmdScope : Scope  NumInputPorts=4
      settings: RequirementInfo={} %GIDa_44f9dfb2_1047_4c85_9993_6df91b14ae0d  YMin=-2~-4~-40~-40  YMax=2~4~40~40  SaveName=ScopeData6
  Integrator1 : Integrator  RequirementInfo={} %GIDa_fc49dfc1_f8ad_44f0_8a9e_cfbd72fa983d  ExternalReset=level  InitialConditionSource=external
  Logical Operator : Logic  RequirementInfo={} %GIDa_a3be1b8e_7e30_4ddb_8576_d6096a49c77e  Operator=NOT  AllPortsSameDT=off  OutDataTypeStr=boolean
  Mux1 : Mux  RequirementInfo={} %GIDa_fa4de243_ff79_4635_bf84_ab68fc6f4471  Inputs=2
  Saturation : Saturate  RequirementInfo={} %GIDa_34361c95_77fe_4878_a89a_f2e2245d083f  UpperLimit=1000  LowerLimit=0.0001
  Saturation Dynamic1 : simulink/Discontinuities/Saturation Dynamic  RequirementInfo={} %GIDa_3c1bb0e4_035b_467b_b908_73d0679fa8c4  OutMin=[]  OutMax=[]  OutDataTypeStr=Inherit: Same as second input  OutDataType=fixdt(1, 16)  OutScaling=2^-10  DoSatur=off
  Sum2 : Sum  RequirementInfo={} %GIDa_0134b7ed_8c9c_449a_ac58_c6bc449e5dc3  Inputs=|+-
  Sum3 : Sum  RequirementInfo={} %GIDa_133a47a4_a1d1_45cf_bb65_a8e707312c61  Inputs=|+-
  Trigonometric Function : Trigonometry  RequirementInfo={} %GIDa_9fedb248_844e_457e_a851_4a39016fb810  Operator=tan
  VarLimIntegIC : Subsystem  RequirementInfo={} %GIDa_5e236912_7c4b_441a_a6c7_d31391da156a
  init : Constant  RequirementInfo={} %GIDa_bb6a6882_f5a4_4f54_8f02_3d74a10327cc  Value=0
  k : Gain  RequirementInfo={} %GIDa_b3adcecb_db12_4f0e_a73c_fd191106ac98  Gain=-1.0
  k1 : Gain  RequirementInfo={} %GIDa_4080639b_e5dd_4b50_81e0_40e346cb6275  Gain=-1.0
  k2 : Gain  RequirementInfo={} %GIDa_3129ff2a_7a94_46f5_a52d_bf604afbaa9d  Gain=1.6878
  k3 : Gain  RequirementInfo={} %GIDa_bc42355c_264a_47e1_8506_c4c4e8e068fc  Gain=pi/180
  k4 : Gain  RequirementInfo={} %GIDa_0e3e2a32_c8b7_428f_ab0c_0faebbbf5e76  Gain=32.174
  k5 : Gain  RequirementInfo={} %GIDa_be5380e6_e279_4fba_b4a2_cea2808c46f4  Gain=180/pi
  k6 : Gain  RequirementInfo={} %GIDa_bccc5425_7281_49cf_93c6_a752e7732049  Gain=2
  omegaSq : Product  RequirementInfo={} %GIDa_e5c95743_58d1_4d7b_8e0f_0d5dca474f7a  RndMeth=Zero
  omegaSq2 : Product  RequirementInfo={} %GIDa_907b30dd_aede_4316_9a8a_044ea704cef8  RndMeth=Zero
  HdgCmd : Outport  RequirementInfo={} %GIDa_7c7f0b37_435d_4e7c_952c_62c879fcb657
  HdgRteCmd : Outport  RequirementInfo={} %GIDa_0b79bbaa_a2da_4cb9_814f_266c555013e7  Port=2
  wires:
  Integrator1/1 -> Sum2/2, HdgCmd/1, HdgCmdScope/3  "HdgCmd"
  Vt/1 -> k2/1
  k2/1 -> Saturation/1  "VTfps"
  Fcn/1 -> omegaSq/2, omegaSq/1, k6/1  "omega"
  k/1 -> Saturation Dynamic1/3
  Mux1/1 -> Fcn2/1
  RollLimit/1 -> k3/1
  Sum3/1 -> Saturation Dynamic1/2  "eaccel"
  Saturation Dynamic1/1 -> VarLimIntegIC/3(In), HdgCmdScope/1  "LimAccel"
  k3/1 -> Trigonometric Function/1
  Trigonometric Function/1 -> k4/1
  k4/1 -> k5/1
  k5/1 -> Mux1/2
  Fcn2/1 -> VarLimIntegIC/1(UpLim), k1/1  "RateLim"
  k1/1 -> VarLimIntegIC/2(LoLim)
  VarLimIntegIC/1(Out) -> Integrator1/1, HdgCmdScope/2, 2zetaOmega/1, HdgRteCmd/1  "LimRate"
  k6/1 -> 2zetaOmega/2
  2zetaOmega/1 -> Sum3/2
  Fcn1/1 -> k/1, Saturation Dynamic1/1
  init/1 -> VarLimIntegIC/5(IC)
  omegaSq/1 -> omegaSq2/1
  omegaSq2/1 -> Sum3/1
  Sum2/1 -> ANGL/1(in)  "epos"
  HdgCmdMCP/1 -> Logical Operator/1, Sum2/1, HdgCmdScope/4  "Cmd"
  ANGL/1(+ -180) -> omegaSq2/2
  Logical Operator/1 -> VarLimIntegIC/4(Trig), Integrator1/2
  Saturation/1 -> Fcn/1, Mux1/1, Fcn1/1
  Heading/1 -> Integrator1/3
